simulink model "gm_AddMul"  (R2021b)
settings: Solver=FixedStepDiscrete  StartTime=0.0  StopTime=10.0  RelTol=1e-3
settings Model: Creator=Student  LastModifiedBy=Student
settings OptimizationCC: BlockReduction=off  ConditionallyExecuteInputs=off  DefaultParameterBehavior=Inlined  InheritOutputTypeSmallerThanSingle=on
settings DebuggingCC: AlgebraicLoopMsg=error  InheritedTsInSrcMsg=none  SingleTaskRateTransMsg=error
settings HardwareCC: ProdBitPerPointer=32  ProdBitPerSizeT=32  ProdBitPerPtrDiffT=32  ProdLargestAtomicFloat=None  ProdIntDivRoundTo=Undefined  ProdEndianess=Unspecified  ProdWordSize=32  ProdHWDeviceType=ASIC/FPGA->ASIC/FPGA  TargetBitPerPointer=64  TargetBitPerSizeT=64  TargetBitPerPtrDiffT=64  TargetLongLongMode=on  TargetIntDivRoundTo=Zero  TargetEndianess=LittleEndian  TargetWordSize=64  TargetHWDeviceType=Custom Processor->MATLAB Host Computer  ProdEqTarget=off

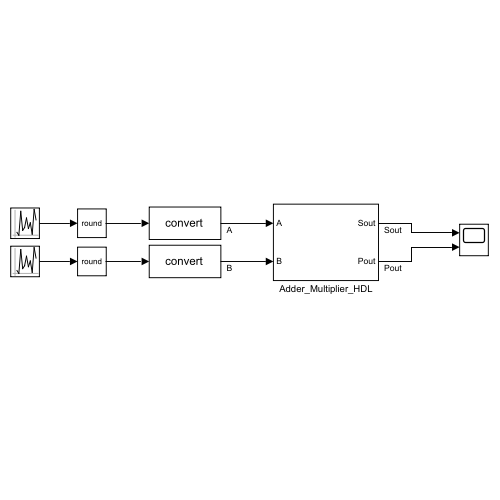
[thumbnail: Simulink's stored preview of the top-level diagram]
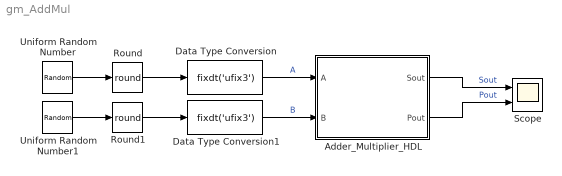
== system gm_AddMul ==
  Adder_Multiplier_HDL : Subsystem
  Data Type Conversion : DataTypeConversion  OutDataTypeStr=fixdt('ufix3')
  Data Type Conversion1 : DataTypeConversion  OutDataTypeStr=fixdt('ufix3')
  Round : Rounding  Operator=round
  Round1 : Rounding  Operator=round
  Scope : Scope  NumInputPorts=2
  Uniform Random Number : UniformRandomNumber  Minimum=0  Maximum=7
  Uniform Random Number1 : UniformRandomNumber  Minimum=0  Maximum=7  Seed=5
  wires:
  Data Type Conversion1/1 -> Adder_Multiplier_HDL/2(B)  "B"
  Uniform Random Number1/1 -> Round1/1
  Round1/1 -> Data Type Conversion1/1
  Data Type Conversion/1 -> Adder_Multiplier_HDL/1(A)  "A"
  Round/1 -> Data Type Conversion/1
  Uniform Random Number/1 -> Round/1
  Adder_Multiplier_HDL/2(Pout) -> Scope/2  "Pout"
  Adder_Multiplier_HDL/1(Sout) -> Scope/1  "Sout"

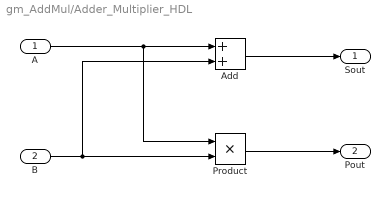
== system gm_AddMul/Adder_Multiplier_HDL ==
  A : Inport
  B : Inport  Port=2
  Add : Sum
  Product : Product
  Sout : Outport
  Pout : Outport  Port=2
  wires:
  Product/1 -> Pout/1
  Add/1 -> Sout/1
  A/1 -> Add/1, Product/1
  B/1 -> Product/2, Add/2
